simulink library "custom_electric_component_library"  (R2018a)
settings: Solver=VariableStepAuto  StartTime=0.0  StopTime=10.0  RelTol=1e-3
values from neighbouring files (symbols this model uses):
  sample_time = 1e-6    (= 1e-06)    [TotemPolePFC_sim.m]
undefined symbols (not defined in the file or in its folder): L_cable, R_cable
libraries: powerlib x14
settings Model: Creator=snow_  LastModifiedBy=snow_

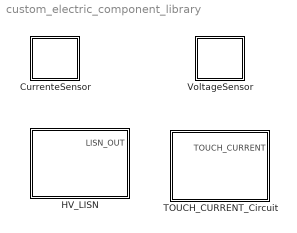
== system custom_electric_component_library ==
  CurrenteSensor : Subsystem  mask{VariableName=Var, SampleTime=1e-6}
      mask prompts: VariableName "Simulink:blkprm_prompts:ToWksVarName"
      settings: AttributesFormatString=%<VariableName>
      mask TypeOptions VariableName: To Workspace1/VariableName | Goto/GotoTag
      mask DialogControl VariableName Prompt: 変数名:
      mask Display:
      | % disp("Current \n Sensor")
      | port_label('lconn', 1, '+')
      | port_label('rconn', 1, '-')
      | 
      | 
      | plot(-50,-35,50,50-15,...
      |     [0,9,18,24,29,30,29,24,18,9,0,-9,-18,-24,-29,-30,-29,-24,-18,-9,0],...
      |     0.8*[30,29,24,18,9,0,-9,-18,-24,-29,-30,-29,-24,-18,-9,0,9,18,24,29,30],...
      |     [-15,0,15],0.8*[-15,25,-15],...
      |     [-7,0,7],0.8*[5,5,5]);
  HV_LISN : Subsystem
  "TOUCH_CURRENT_Circuit " : Subsystem
  VoltageSensor : Subsystem  mask{VariableName=Var, SampleTime=1e-6}
      mask prompts: VariableName "Simulink:blkprm_prompts:ToWksVarName"
      settings: AttributesFormatString=%<VariableName>
      mask TypeOptions VariableName: To Workspace1/VariableName | Goto/GotoTag
      mask DialogControl VariableName Prompt: 変数名:
      mask Display:
      | %disp("Voltage \n Sensor")
      | port_label('lconn', 1, '+')
      | port_label('lconn', 2, '-')
      | 
      | plot(-50,-35,50,50-15,...
      |     [0,9,18,24,29,30,29,24,18,9,0,-9,-18,-24,-29,-30,-29,-24,-18,-9,0],...
      |     0.8*[30,29,24,18,9,0,-9,-18,-24,-29,-30,-29,-24,-18,-9,0,9,18,24,29,30],...
      |     [-15,0,15],0.8*[15,-20,15]);

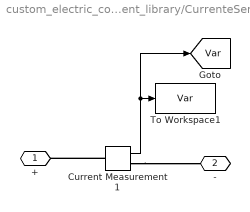
== system custom_electric_component_library/CurrenteSensor ==
  Current Measurement1 : powerlib/Measurements/Current Measurement  PhasorSimulation=off  OutputType=Complex  PSBequivalent=0
  To Workspace1 : ToWorkspace  VariableName=Var  SampleTime=sample_time
  + : PMIOPort  Side=Left
  - : PMIOPort  Port=2  Side=Right
  tag scope: Var=global
  wires:
  Current Measurement1/1 -> [Var], To Workspace1/1
  connections:
  Current Measurement1/LConn1 -- +/RConn1
  Current Measurement1/RConn1 -- -/RConn1

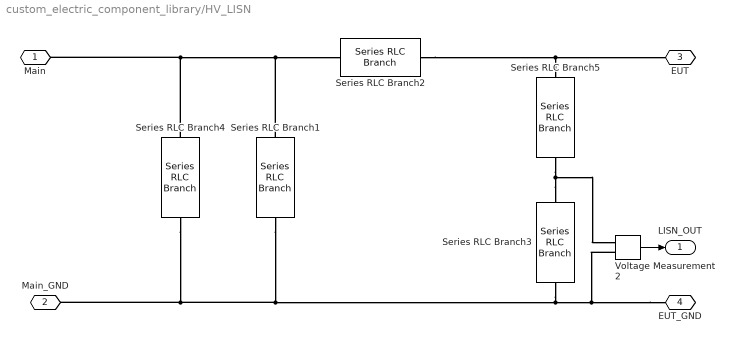
== system custom_electric_component_library/HV_LISN ==
  Series RLC Branch1 : powerlib/Elements/Series RLC Branch  LConnTagsString=__new0  RConnTagsString=__new0  BranchType=C  Resistance=24e-3  Inductance=1000e-6  SetiL0=off  InitialCurrent=0  Capacitance=0.1e-6  Setx0=off  InitialVoltage=0  Measurements=None
      settings: AttributesFormatString="C= %<Capacitance>  F"
  Series RLC Branch2 : powerlib/Elements/Series RLC Branch  LConnTagsString=__new0  RConnTagsString=__new0  BranchType=L  Resistance=R_cable  Inductance=5e-6  SetiL0=off  InitialCurrent=0  Capacitance=1e-6  Setx0=off  InitialVoltage=0  Measurements=None
      settings: AttributesFormatString=L=%<Inductance> H
  Series RLC Branch3 : powerlib/Elements/Series RLC Branch  LConnTagsString=__new0  RConnTagsString=__new0  BranchType=R  Resistance=1e3  Inductance=L_cable  SetiL0=off  InitialCurrent=0  Capacitance=1e-6  Setx0=off  InitialVoltage=0  Measurements=None
      settings: AttributesFormatString=R=%<Resistance> Ohm
  Series RLC Branch4 : powerlib/Elements/Series RLC Branch  LConnTagsString=__new0  RConnTagsString=__new0  BranchType=R  Resistance=1e6  Inductance=L_cable  SetiL0=off  InitialCurrent=0  Capacitance=1e-6  Setx0=off  InitialVoltage=0  Measurements=None
      settings: AttributesFormatString=R=%<Resistance> Ohm
  Series RLC Branch5 : powerlib/Elements/Series RLC Branch  LConnTagsString=__new0  RConnTagsString=__new0  BranchType=C  Resistance=24e-3  Inductance=1000e-6  SetiL0=off  InitialCurrent=0  Capacitance=0.1e-6  Setx0=off  InitialVoltage=0  Measurements=None
      settings: AttributesFormatString="C= %<Capacitance>  F"
  Voltage Measurement2 : powerlib/Measurements/Voltage Measurement  PhasorSimulation=off  OutputType=Complex  PSBequivalent=0
  Main : PMIOPort  Side=Left
  Main_GND : PMIOPort  Port=2  Side=Left
  EUT : PMIOPort  Port=3  Side=Right
  EUT_GND : PMIOPort  Port=4  Side=Right
  LISN_OUT : Outport
  wires:
  Voltage Measurement2/1 -> LISN_OUT/1
  connections:
  EUT_GND/RConn1 -- Series RLC Branch1/RConn1 -- Series RLC Branch4/RConn1 -- Main_GND/RConn1 -- Series RLC Branch3/RConn1 -- Voltage Measurement2/LConn2
  Series RLC Branch1/LConn1 -- Series RLC Branch2/LConn1 -- Series RLC Branch4/LConn1 -- Main/RConn1
  Series RLC Branch3/LConn1 -- Series RLC Branch5/RConn1 -- Voltage Measurement2/LConn1
  Series RLC Branch2/RConn1 -- EUT/RConn1 -- Series RLC Branch5/LConn1

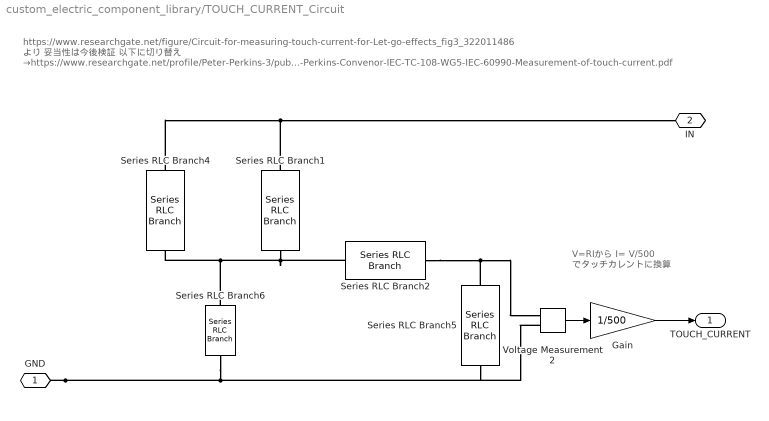
== system custom_electric_component_library/TOUCH_CURRENT_Circuit  ==
  note: V=RIから
      | 　I=　V/500 でタッチカレントに換算
  note: https://www.researchgate.net/figure/Circuit-for-measuring-touch-current-for-Let-go-effects_fig3_322011486 より
      | 妥当性は今後検証
      | 以下に切り替え
      | →https://www.researchgate.net/profile/Peter-Perkins-3/publication/299508095_IEC_60990_Touch_Current_circuits_Component_tolerance_analysis_Peter_E_Perkins_Convenor_IEC_TC_108WG5_'IEC_60990_Measurement_of_touch_current_'/links/56fc7f7408ae8239f6dc4a67/IEC-60990-Touch-Current-circuits-Component-tolerance-analysis-Peter-E-Perkins-Convenor-IEC-TC-108-WG5-IEC-60990-Measurement-of-touch-current.pdf
  Gain : Gain  Gain=1/500
  Series RLC Branch1 : powerlib/Elements/Series RLC Branch  LConnTagsString=__new0  RConnTagsString=__new0  BranchType=C  Resistance=24e-3  Inductance=1000e-6  SetiL0=off  InitialCurrent=0  Capacitance=0.22e-6  Setx0=off  InitialVoltage=0  Measurements=None
      settings: AttributesFormatString="C= %<Capacitance>  F"
  Series RLC Branch2 : powerlib/Elements/Series RLC Branch  LConnTagsString=__new0  RConnTagsString=__new0  BranchType=R  Resistance=10e3  Inductance=L_cable  SetiL0=off  InitialCurrent=0  Capacitance=1e-6  Setx0=off  InitialVoltage=0  Measurements=None
      settings: AttributesFormatString=R=%<Resistance> Ohm
  Series RLC Branch4 : powerlib/Elements/Series RLC Branch  LConnTagsString=__new0  RConnTagsString=__new0  BranchType=R  Resistance=1500  Inductance=L_cable  SetiL0=off  InitialCurrent=0  Capacitance=1e-6  Setx0=off  InitialVoltage=0  Measurements=None
      settings: AttributesFormatString=R=%<Resistance> Ohm
  Series RLC Branch5 : powerlib/Elements/Series RLC Branch  LConnTagsString=__new0  RConnTagsString=__new0  BranchType=C  Resistance=24e-3  Inductance=1000e-6  SetiL0=off  InitialCurrent=0  Capacitance=0.022e-6  Setx0=off  InitialVoltage=0  Measurements=None
      settings: AttributesFormatString="C= %<Capacitance>  F"
  Series RLC Branch6 : powerlib/Elements/Series RLC Branch  LConnTagsString=__new0  RConnTagsString=__new0  BranchType=R  Resistance=500  Inductance=L_cable  SetiL0=off  InitialCurrent=0  Capacitance=1e-6  Setx0=off  InitialVoltage=0  Measurements=None
      settings: AttributesFormatString=R=%<Resistance> Ohm
  Voltage Measurement2 : powerlib/Measurements/Voltage Measurement  PhasorSimulation=off  OutputType=Complex  PSBequivalent=0
  GND : PMIOPort  Side=Left
  IN : PMIOPort  Port=2  Side=Right
  TOUCH_CURRENT : Outport
  wires:
  Voltage Measurement2/1 -> Gain/1
  Gain/1 -> TOUCH_CURRENT/1
  connections:
  GND/RConn1 -- Series RLC Branch6/RConn1 -- Series RLC Branch5/RConn1 -- Voltage Measurement2/LConn2
  Series RLC Branch5/LConn1 -- Series RLC Branch2/RConn1 -- Voltage Measurement2/LConn1
  Series RLC Branch4/LConn1 -- Series RLC Branch1/LConn1 -- IN/RConn1
  Series RLC Branch2/LConn1 -- Series RLC Branch1/RConn1 -- Series RLC Branch6/LConn1 -- Series RLC Branch4/RConn1

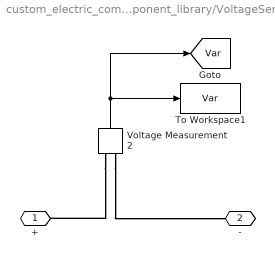
== system custom_electric_component_library/VoltageSensor ==
  To Workspace1 : ToWorkspace  VariableName=Var  SampleTime=SampleTime
  Voltage Measurement2 : powerlib/Measurements/Voltage Measurement  PhasorSimulation=off  OutputType=Complex  PSBequivalent=0
  + : PMIOPort  Side=Left
  - : PMIOPort  Port=2  Side=Left
  tag scope: Var=global
  wires:
  Voltage Measurement2/1 -> [Var], To Workspace1/1
  connections:
  Voltage Measurement2/LConn1 -- +/RConn1
  Voltage Measurement2/LConn2 -- -/RConn1
